simulink model "IIR4_int_quant"  (R2016b)
settings: Solver=VariableStepAuto  StartTime=0.0  StopTime=10.0  RelTol=1e-3
libraries: dspstat3 x2
settings Model: Creator=biren  LastModifiedBy=biren

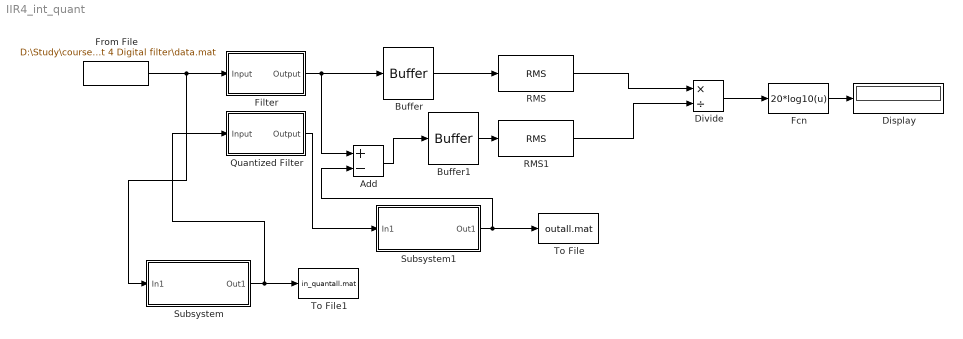
== system IIR4_int_quant ==
  Add : Sum  Inputs=+-
  Buffer : Buffer  TreatMby1Signals=One channel  OutputFrames=off
  Buffer1 : Buffer  TreatMby1Signals=One channel  OutputFrames=off
  Display : Display
  Divide : Product  Inputs=*/
  Fcn : Fcn  Expr=20*log10(u)
  "Filter " : Subsystem  Tag=FilterWizardSubSystem
      settings: ErrorFcn=dspFilterRealizedInBasicElemsAlgLoopErrFcnCallback
  From File : FromFile  FileName=D:\Study\courses\ECEN654\Assignment 4 Digital filter\data.mat  SampleTime=1/44100
  Quantized Filter : Subsystem  Tag=FilterWizardSubSystem  mask{ck=11}
      settings: ErrorFcn=dspFilterRealizedInBasicElemsAlgLoopErrFcnCallback
  RMS : dspstat3/RMS  run=off  directionMode=Each column  dimension=1  InputProcessing=Columns as channels (frame based)  reset_popup=None
  RMS1 : dspstat3/RMS  run=off  directionMode=Each column  dimension=1  InputProcessing=Columns as channels (frame based)  reset_popup=None
  Subsystem : Subsystem  mask{k=12, s=5}
  Subsystem1 : Subsystem  mask{k=12, s=5}
  To File : ToFile  Filename=outall.mat
  To File1 : ToFile  Filename=in_quantall.mat
  wires:
  "Filter "/1(Output) -> Buffer/1, Add/1
  Add/1 -> Buffer1/1
  Buffer/1 -> RMS/1
  Buffer1/1 -> RMS1/1
  Subsystem1/1(Out1) -> To File/1, Add/2
  Subsystem/1(Out1) -> To File1/1, Quantized Filter/1(Input)
  From File/1 -> Subsystem/1(In1), "Filter "/1(Input)
  RMS/1 -> Divide/1
  RMS1/1 -> Divide/2
  Divide/1 -> Fcn/1
  Fcn/1 -> Display/1
  Quantized Filter/1(Output) -> Subsystem1/1(In1)

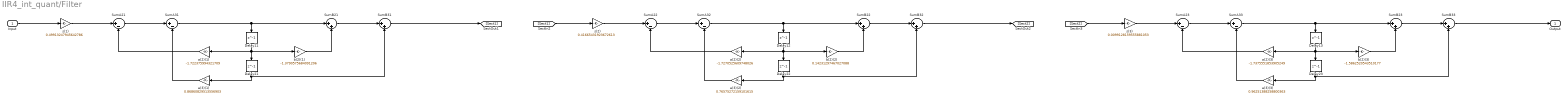
== system IIR4_int_quant/Filter  ==
  Input : Inport
  Delay{11..13,21..23} (6 alike) : Delay  DelayLength=1  InitialCondition=0
  SumA{21..23,31..33} (6 alike) : Sum  Inputs=|+-  RndMeth=Nearest  SaturateOnIntegerOverflow=on  OutDataTypeStr=Inherit: Same as first input
  SumB{21..23,31..33} (6 alike) : Sum  Inputs=|++  RndMeth=Nearest  SaturateOnIntegerOverflow=on  OutDataTypeStr=Inherit: Same as first input
  a(2)(1) : Gain  Gain=-1.722375994321709  ParamDataTypeStr=double  RndMeth=Nearest  SaturateOnIntegerOverflow=on  OutDataTypeStr=Inherit: Same as input
  a(2)(2) : Gain  Gain=-1.7270525609748026  ParamDataTypeStr=double  RndMeth=Nearest  SaturateOnIntegerOverflow=on  OutDataTypeStr=Inherit: Same as input
  a(2)(3) : Gain  Gain=-1.7375551853905249  ParamDataTypeStr=double  RndMeth=Nearest  SaturateOnIntegerOverflow=on  OutDataTypeStr=Inherit: Same as input
  a(3)(1) : Gain  Gain=0.86860829513556903  ParamDataTypeStr=double  RndMeth=Nearest  SaturateOnIntegerOverflow=on  OutDataTypeStr=Inherit: Same as input
  a(3)(2) : Gain  Gain=0.76575272159101615  ParamDataTypeStr=double  RndMeth=Nearest  SaturateOnIntegerOverflow=on  OutDataTypeStr=Inherit: Same as input
  a(3)(3) : Gain  Gain=0.96251388258800363  ParamDataTypeStr=double  RndMeth=Nearest  SaturateOnIntegerOverflow=on  OutDataTypeStr=Inherit: Same as input
  b(2)(1) : Gain  Gain=-1.3790575684091206  ParamDataTypeStr=double  RndMeth=Nearest  SaturateOnIntegerOverflow=on  OutDataTypeStr=Inherit: Same as input
  b(2)(2) : Gain  Gain=0.14231297467027088  ParamDataTypeStr=double  RndMeth=Nearest  SaturateOnIntegerOverflow=on  OutDataTypeStr=Inherit: Same as input
  b(2)(3) : Gain  Gain=-1.5862520543510177  ParamDataTypeStr=double  RndMeth=Nearest  SaturateOnIntegerOverflow=on  OutDataTypeStr=Inherit: Same as input
  s(1) : Gain  Gain=0.49913247945642786  ParamDataTypeStr=double  RndMeth=Nearest  SaturateOnIntegerOverflow=on  OutDataTypeStr=Inherit: Same as input
  s(2) : Gain  Gain=0.41665431923672613  ParamDataTypeStr=double  RndMeth=Nearest  SaturateOnIntegerOverflow=on  OutDataTypeStr=Inherit: Same as input
  s(3) : Gain  Gain=0.0099128159555881053  ParamDataTypeStr=double  RndMeth=Nearest  SaturateOnIntegerOverflow=on  OutDataTypeStr=Inherit: Same as input
  Output : Outport
  wires:
  Input/1 -> s(1)/1
  s(1)/1 -> SumA21/1
  SumA21/1 -> SumA31/1
  SumA31/1 -> SumB21/1, Delay11/1
  SumB21/1 -> SumB31/1
  SumB31/1 -> [Sect1]
  a(2)(1)/1 -> SumA21/2
  Delay11/1 -> a(2)(1)/1, b(2)(1)/1, Delay21/1
  b(2)(1)/1 -> SumB21/2
  a(3)(1)/1 -> SumA31/2
  Delay21/1 -> a(3)(1)/1, SumB31/2
  [Sect1] -> s(2)/1
  s(2)/1 -> SumA22/1
  SumA22/1 -> SumA32/1
  SumA32/1 -> SumB22/1, Delay12/1
  SumB22/1 -> SumB32/1
  SumB32/1 -> [Sect2]
  a(2)(2)/1 -> SumA22/2
  Delay12/1 -> a(2)(2)/1, b(2)(2)/1, Delay22/1
  b(2)(2)/1 -> SumB22/2
  a(3)(2)/1 -> SumA32/2
  Delay22/1 -> a(3)(2)/1, SumB32/2
  [Sect2] -> s(3)/1
  s(3)/1 -> SumA23/1
  SumA23/1 -> SumA33/1
  SumA33/1 -> SumB23/1, Delay13/1
  SumB23/1 -> SumB33/1
  SumB33/1 -> Output/1
  a(2)(3)/1 -> SumA23/2
  Delay13/1 -> a(2)(3)/1, b(2)(3)/1, Delay23/1
  b(2)(3)/1 -> SumB23/2
  a(3)(3)/1 -> SumA33/2
  Delay23/1 -> a(3)(3)/1, SumB33/2

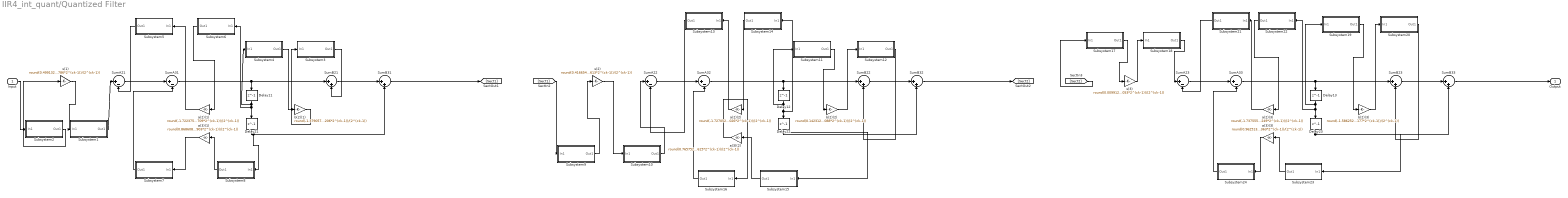
== system IIR4_int_quant/Quantized Filter ==
  Input : Inport
  Delay{11..13,21..23} (6 alike) : Delay  DelayLength=1  InitialCondition=0
  Subsystem1 : Subsystem  mask{k=12, s=5}
  Subsystem10 : Subsystem  mask{k=12, s=5}
  Subsystem11 : Subsystem  mask{k=12, s=5}
  Subsystem12 : Subsystem  mask{k=12, s=5}
  Subsystem13 : Subsystem  mask{k=12, s=5}
  Subsystem14 : Subsystem  mask{k=12, s=5}
  Subsystem15 : Subsystem  mask{k=12, s=5}
  Subsystem16 : Subsystem  mask{k=12, s=5}
  Subsystem17 : Subsystem  mask{k=12, s=5}
  Subsystem18 : Subsystem  mask{k=12, s=5}
  Subsystem19 : Subsystem  mask{k=12, s=5}
  Subsystem2 : Subsystem  mask{k=12, s=5}
  Subsystem20 : Subsystem  mask{k=12, s=5}
  Subsystem21 : Subsystem  mask{k=12, s=5}
  Subsystem22 : Subsystem  mask{k=12, s=5}
  Subsystem23 : Subsystem  mask{k=12, s=5}
  Subsystem24 : Subsystem  mask{k=12, s=5}
  Subsystem3 : Subsystem  mask{k=12, s=5}
  Subsystem4 : Subsystem  mask{k=12, s=5}
  Subsystem5 : Subsystem  mask{k=12, s=5}
  Subsystem6 : Subsystem  mask{k=12, s=5}
  Subsystem7 : Subsystem  mask{k=12, s=5}
  Subsystem8 : Subsystem  mask{k=12, s=5}
  Subsystem9 : Subsystem  mask{k=12, s=5}
  SumA{21..23,31..33} (6 alike) : Sum  Inputs=|+-  RndMeth=Nearest  SaturateOnIntegerOverflow=on  OutDataTypeStr=Inherit: Same as first input
  SumB{21..23,31..33} (6 alike) : Sum  Inputs=|++  RndMeth=Nearest  SaturateOnIntegerOverflow=on  OutDataTypeStr=Inherit: Same as first input
  a(2)(1) : Gain  Gain=round(-1.722375994321709*2^(ck-1))/(2^(ck-1))  ParamDataTypeStr=double  RndMeth=Nearest  SaturateOnIntegerOverflow=on  OutDataTypeStr=Inherit: Same as input
  a(2)(2) : Gain  Gain=round(-1.7270525609748026*2^(ck-1))/(2^(ck-1))  ParamDataTypeStr=double  RndMeth=Nearest  SaturateOnIntegerOverflow=on  OutDataTypeStr=Inherit: Same as input
  a(2)(3) : Gain  Gain=round(-1.7375551853905249*2^(ck-1))/(2^(ck-1))  ParamDataTypeStr=double  RndMeth=Nearest  SaturateOnIntegerOverflow=on  OutDataTypeStr=Inherit: Same as input
  a(3)(1) : Gain  Gain=round(0.86860829513556903*2^(ck-1))/(2^(ck-1))  ParamDataTypeStr=double  RndMeth=Nearest  SaturateOnIntegerOverflow=on  OutDataTypeStr=Inherit: Same as input
  a(3)(2) : Gain  Gain=round(0.76575272159101615*2^(ck-1))/(2^(ck-1))  ParamDataTypeStr=double  RndMeth=Nearest  SaturateOnIntegerOverflow=on  OutDataTypeStr=Inherit: Same as input
  a(3)(3) : Gain  Gain=round(0.96251388258800363*2^(ck-1))/(2^(ck-1))  ParamDataTypeStr=double  RndMeth=Nearest  SaturateOnIntegerOverflow=on  OutDataTypeStr=Inherit: Same as input
  b(2)(1) : Gain  Gain=round(-1.3790575684091206*2^(ck-1))/(2^(ck-1))  ParamDataTypeStr=double  RndMeth=Nearest  SaturateOnIntegerOverflow=on  OutDataTypeStr=Inherit: Same as input
  b(2)(2) : Gain  Gain=round(0.14231297467027088*2^(ck-1))/(2^(ck-1))  ParamDataTypeStr=double  RndMeth=Nearest  SaturateOnIntegerOverflow=on  OutDataTypeStr=Inherit: Same as input
  b(2)(3) : Gain  Gain=round(-1.5862520543510177*2^(ck-1))/(2^(ck-1))  ParamDataTypeStr=double  RndMeth=Nearest  SaturateOnIntegerOverflow=on  OutDataTypeStr=Inherit: Same as input
  s(1) : Gain  Gain=round(0.49913247945642786*2^(ck-1))/(2^(ck-1))  ParamDataTypeStr=double  RndMeth=Nearest  SaturateOnIntegerOverflow=on  OutDataTypeStr=Inherit: Same as input
  s(2) : Gain  Gain=round(0.41665431923672613*2^(ck-1))/(2^(ck-1))  ParamDataTypeStr=double  RndMeth=Nearest  SaturateOnIntegerOverflow=on  OutDataTypeStr=Inherit: Same as input
  s(3) : Gain  Gain=round(0.0099128159555881053*2^(ck-1))/(2^(ck-1))  ParamDataTypeStr=double  RndMeth=Nearest  SaturateOnIntegerOverflow=on  OutDataTypeStr=Inherit: Same as input
  Output : Outport
  wires:
  SumA21/1 -> SumA31/1
  SumA31/1 -> SumB21/1, Delay11/1
  SumB21/1 -> SumB31/1
  SumB31/1 -> [Sect1]
  Delay11/1 -> Subsystem4/1(In1), Subsystem6/1(In1), Delay21/1
  Delay21/1 -> Subsystem8/1(In1), SumB31/2
  SumA22/1 -> SumA32/1
  SumA32/1 -> SumB22/1, Delay12/1
  SumB22/1 -> SumB32/1
  SumB32/1 -> [Sect2]
  Delay12/1 -> Subsystem11/1(In1), Subsystem14/1(In1), Delay22/1
  Delay22/1 -> Subsystem15/1(In1), SumB32/2
  SumA23/1 -> SumA33/1
  SumA33/1 -> SumB23/1, Delay13/1
  SumB23/1 -> SumB33/1
  SumB33/1 -> Output/1
  Delay13/1 -> Subsystem19/1(In1), Subsystem22/1(In1), Delay23/1
  Delay23/1 -> Subsystem23/1(In1), SumB33/2
  s(1)/1 -> Subsystem1/1(In1)
  Subsystem1/1(Out1) -> SumA21/1
  Input/1 -> Subsystem2/1(In1)
  Subsystem2/1(Out1) -> s(1)/1
  Subsystem4/1(Out1) -> b(2)(1)/1
  b(2)(1)/1 -> Subsystem3/1(In1)
  Subsystem3/1(Out1) -> SumB21/2
  Subsystem6/1(Out1) -> a(2)(1)/1
  a(2)(1)/1 -> Subsystem5/1(In1)
  Subsystem5/1(Out1) -> SumA21/2
  Subsystem8/1(Out1) -> a(3)(1)/1
  a(3)(1)/1 -> Subsystem7/1(In1)
  Subsystem7/1(Out1) -> SumA31/2
  [Sect1] -> Subsystem9/1(In1)
  Subsystem9/1(Out1) -> s(2)/1
  s(2)/1 -> Subsystem10/1(In1)
  Subsystem10/1(Out1) -> SumA22/1
  Subsystem11/1(Out1) -> b(2)(2)/1
  b(2)(2)/1 -> Subsystem12/1(In1)
  Subsystem12/1(Out1) -> SumB22/2
  Subsystem14/1(Out1) -> a(2)(2)/1
  a(2)(2)/1 -> Subsystem13/1(In1)
  Subsystem13/1(Out1) -> SumA22/2
  Subsystem15/1(Out1) -> a(3)(2)/1
  a(3)(2)/1 -> Subsystem16/1(In1)
  Subsystem16/1(Out1) -> SumA32/2
  [Sect2] -> Subsystem17/1(In1)
  Subsystem17/1(Out1) -> s(3)/1
  s(3)/1 -> Subsystem18/1(In1)
  Subsystem18/1(Out1) -> SumA23/1
  Subsystem19/1(Out1) -> b(2)(3)/1
  b(2)(3)/1 -> Subsystem20/1(In1)
  Subsystem20/1(Out1) -> SumB23/2
  Subsystem22/1(Out1) -> a(2)(3)/1
  a(2)(3)/1 -> Subsystem21/1(In1)
  Subsystem21/1(Out1) -> SumA23/2
  Subsystem23/1(Out1) -> a(3)(3)/1
  Subsystem24/1(Out1) -> SumA33/2
  a(3)(3)/1 -> Subsystem24/1(In1)

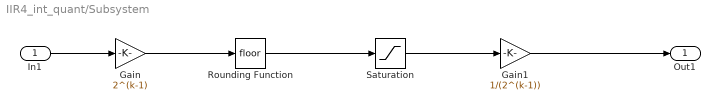
== system IIR4_int_quant/Subsystem ==
  In1 : Inport
  Gain : Gain  Gain=2^(k-1)
  Gain1 : Gain  Gain=1/(2^(k-1))
  Rounding Function : Rounding
  Saturation : Saturate  UpperLimit=2^(k+s-1) - 1  LowerLimit=-2^(k+s-1)
  Out1 : Outport
  wires:
  In1/1 -> Gain/1
  Gain/1 -> Rounding Function/1
  Rounding Function/1 -> Saturation/1
  Saturation/1 -> Gain1/1
  Gain1/1 -> Out1/1

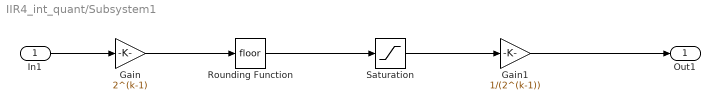
== system IIR4_int_quant/Subsystem1 ==
  In1 : Inport
  Gain : Gain  Gain=2^(k-1)
  Gain1 : Gain  Gain=1/(2^(k-1))
  Rounding Function : Rounding
  Saturation : Saturate  UpperLimit=2^(k+s-1) - 1  LowerLimit=-2^(k+s-1)
  Out1 : Outport
  wires:
  In1/1 -> Gain/1
  Gain/1 -> Rounding Function/1
  Rounding Function/1 -> Saturation/1
  Saturation/1 -> Gain1/1
  Gain1/1 -> Out1/1

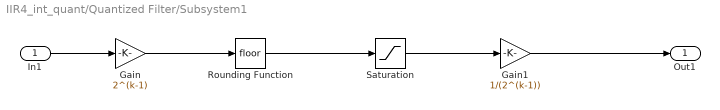
== system IIR4_int_quant/Quantized Filter/Subsystem1 ==
  In1 : Inport
  Gain : Gain  Gain=2^(k-1)
  Gain1 : Gain  Gain=1/(2^(k-1))
  Rounding Function : Rounding
  Saturation : Saturate  UpperLimit=2^(k+s-1) - 1  LowerLimit=-2^(k+s-1)
  Out1 : Outport
  wires:
  In1/1 -> Gain/1
  Gain/1 -> Rounding Function/1
  Rounding Function/1 -> Saturation/1
  Saturation/1 -> Gain1/1
  Gain1/1 -> Out1/1

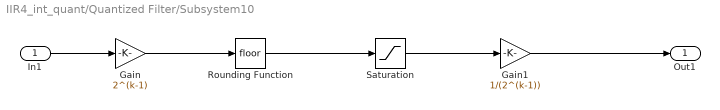
== system IIR4_int_quant/Quantized Filter/Subsystem10 ==
  In1 : Inport
  Gain : Gain  Gain=2^(k-1)
  Gain1 : Gain  Gain=1/(2^(k-1))
  Rounding Function : Rounding
  Saturation : Saturate  UpperLimit=2^(k+s-1) - 1  LowerLimit=-2^(k+s-1)
  Out1 : Outport
  wires:
  In1/1 -> Gain/1
  Gain/1 -> Rounding Function/1
  Rounding Function/1 -> Saturation/1
  Saturation/1 -> Gain1/1
  Gain1/1 -> Out1/1

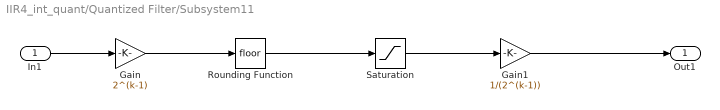
== system IIR4_int_quant/Quantized Filter/Subsystem11 ==
  In1 : Inport
  Gain : Gain  Gain=2^(k-1)
  Gain1 : Gain  Gain=1/(2^(k-1))
  Rounding Function : Rounding
  Saturation : Saturate  UpperLimit=2^(k+s-1) - 1  LowerLimit=-2^(k+s-1)
  Out1 : Outport
  wires:
  In1/1 -> Gain/1
  Gain/1 -> Rounding Function/1
  Rounding Function/1 -> Saturation/1
  Saturation/1 -> Gain1/1
  Gain1/1 -> Out1/1

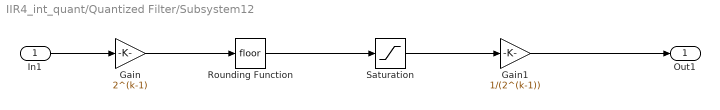
== system IIR4_int_quant/Quantized Filter/Subsystem12 ==
  In1 : Inport
  Gain : Gain  Gain=2^(k-1)
  Gain1 : Gain  Gain=1/(2^(k-1))
  Rounding Function : Rounding
  Saturation : Saturate  UpperLimit=2^(k+s-1) - 1  LowerLimit=-2^(k+s-1)
  Out1 : Outport
  wires:
  In1/1 -> Gain/1
  Gain/1 -> Rounding Function/1
  Rounding Function/1 -> Saturation/1
  Saturation/1 -> Gain1/1
  Gain1/1 -> Out1/1

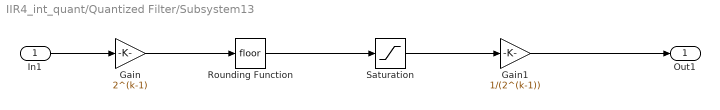
== system IIR4_int_quant/Quantized Filter/Subsystem13 ==
  In1 : Inport
  Gain : Gain  Gain=2^(k-1)
  Gain1 : Gain  Gain=1/(2^(k-1))
  Rounding Function : Rounding
  Saturation : Saturate  UpperLimit=2^(k+s-1) - 1  LowerLimit=-2^(k+s-1)
  Out1 : Outport
  wires:
  In1/1 -> Gain/1
  Gain/1 -> Rounding Function/1
  Rounding Function/1 -> Saturation/1
  Saturation/1 -> Gain1/1
  Gain1/1 -> Out1/1

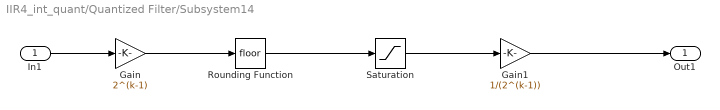
== system IIR4_int_quant/Quantized Filter/Subsystem14 ==
  In1 : Inport
  Gain : Gain  Gain=2^(k-1)
  Gain1 : Gain  Gain=1/(2^(k-1))
  Rounding Function : Rounding
  Saturation : Saturate  UpperLimit=2^(k+s-1) - 1  LowerLimit=-2^(k+s-1)
  Out1 : Outport
  wires:
  In1/1 -> Gain/1
  Gain/1 -> Rounding Function/1
  Rounding Function/1 -> Saturation/1
  Saturation/1 -> Gain1/1
  Gain1/1 -> Out1/1

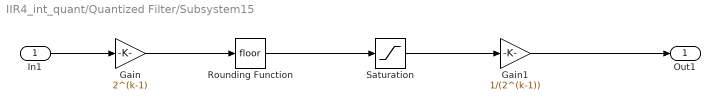
== system IIR4_int_quant/Quantized Filter/Subsystem15 ==
  In1 : Inport
  Gain : Gain  Gain=2^(k-1)
  Gain1 : Gain  Gain=1/(2^(k-1))
  Rounding Function : Rounding
  Saturation : Saturate  UpperLimit=2^(k+s-1) - 1  LowerLimit=-2^(k+s-1)
  Out1 : Outport
  wires:
  In1/1 -> Gain/1
  Gain/1 -> Rounding Function/1
  Rounding Function/1 -> Saturation/1
  Saturation/1 -> Gain1/1
  Gain1/1 -> Out1/1

== system IIR4_int_quant/Quantized Filter/Subsystem16 ==
  In1 : Inport
  Gain : Gain  Gain=2^(k-1)
  Gain1 : Gain  Gain=1/(2^(k-1))
  Rounding Function : Rounding
  Saturation : Saturate  UpperLimit=2^(k+s-1) - 1  LowerLimit=-2^(k+s-1)
  Out1 : Outport
  wires:
  In1/1 -> Gain/1
  Gain/1 -> Rounding Function/1
  Rounding Function/1 -> Saturation/1
  Saturation/1 -> Gain1/1
  Gain1/1 -> Out1/1

== system IIR4_int_quant/Quantized Filter/Subsystem17 ==
  In1 : Inport
  Gain : Gain  Gain=2^(k-1)
  Gain1 : Gain  Gain=1/(2^(k-1))
  Rounding Function : Rounding
  Saturation : Saturate  UpperLimit=2^(k+s-1) - 1  LowerLimit=-2^(k+s-1)
  Out1 : Outport
  wires:
  In1/1 -> Gain/1
  Gain/1 -> Rounding Function/1
  Rounding Function/1 -> Saturation/1
  Saturation/1 -> Gain1/1
  Gain1/1 -> Out1/1

== system IIR4_int_quant/Quantized Filter/Subsystem18 ==
  In1 : Inport
  Gain : Gain  Gain=2^(k-1)
  Gain1 : Gain  Gain=1/(2^(k-1))
  Rounding Function : Rounding
  Saturation : Saturate  UpperLimit=2^(k+s-1) - 1  LowerLimit=-2^(k+s-1)
  Out1 : Outport
  wires:
  In1/1 -> Gain/1
  Gain/1 -> Rounding Function/1
  Rounding Function/1 -> Saturation/1
  Saturation/1 -> Gain1/1
  Gain1/1 -> Out1/1

== system IIR4_int_quant/Quantized Filter/Subsystem19 ==
  In1 : Inport
  Gain : Gain  Gain=2^(k-1)
  Gain1 : Gain  Gain=1/(2^(k-1))
  Rounding Function : Rounding
  Saturation : Saturate  UpperLimit=2^(k+s-1) - 1  LowerLimit=-2^(k+s-1)
  Out1 : Outport
  wires:
  In1/1 -> Gain/1
  Gain/1 -> Rounding Function/1
  Rounding Function/1 -> Saturation/1
  Saturation/1 -> Gain1/1
  Gain1/1 -> Out1/1

== system IIR4_int_quant/Quantized Filter/Subsystem2 ==
  In1 : Inport
  Gain : Gain  Gain=2^(k-1)
  Gain1 : Gain  Gain=1/(2^(k-1))
  Rounding Function : Rounding
  Saturation : Saturate  UpperLimit=2^(k+s-1) - 1  LowerLimit=-2^(k+s-1)
  Out1 : Outport
  wires:
  In1/1 -> Gain/1
  Gain/1 -> Rounding Function/1
  Rounding Function/1 -> Saturation/1
  Saturation/1 -> Gain1/1
  Gain1/1 -> Out1/1

== system IIR4_int_quant/Quantized Filter/Subsystem20 ==
  In1 : Inport
  Gain : Gain  Gain=2^(k-1)
  Gain1 : Gain  Gain=1/(2^(k-1))
  Rounding Function : Rounding
  Saturation : Saturate  UpperLimit=2^(k+s-1) - 1  LowerLimit=-2^(k+s-1)
  Out1 : Outport
  wires:
  In1/1 -> Gain/1
  Gain/1 -> Rounding Function/1
  Rounding Function/1 -> Saturation/1
  Saturation/1 -> Gain1/1
  Gain1/1 -> Out1/1

== system IIR4_int_quant/Quantized Filter/Subsystem21 ==
  In1 : Inport
  Gain : Gain  Gain=2^(k-1)
  Gain1 : Gain  Gain=1/(2^(k-1))
  Rounding Function : Rounding
  Saturation : Saturate  UpperLimit=2^(k+s-1) - 1  LowerLimit=-2^(k+s-1)
  Out1 : Outport
  wires:
  In1/1 -> Gain/1
  Gain/1 -> Rounding Function/1
  Rounding Function/1 -> Saturation/1
  Saturation/1 -> Gain1/1
  Gain1/1 -> Out1/1

== system IIR4_int_quant/Quantized Filter/Subsystem22 ==
  In1 : Inport
  Gain : Gain  Gain=2^(k-1)
  Gain1 : Gain  Gain=1/(2^(k-1))
  Rounding Function : Rounding
  Saturation : Saturate  UpperLimit=2^(k+s-1) - 1  LowerLimit=-2^(k+s-1)
  Out1 : Outport
  wires:
  In1/1 -> Gain/1
  Gain/1 -> Rounding Function/1
  Rounding Function/1 -> Saturation/1
  Saturation/1 -> Gain1/1
  Gain1/1 -> Out1/1

== system IIR4_int_quant/Quantized Filter/Subsystem23 ==
  In1 : Inport
  Gain : Gain  Gain=2^(k-1)
  Gain1 : Gain  Gain=1/(2^(k-1))
  Rounding Function : Rounding
  Saturation : Saturate  UpperLimit=2^(k+s-1) - 1  LowerLimit=-2^(k+s-1)
  Out1 : Outport
  wires:
  In1/1 -> Gain/1
  Gain/1 -> Rounding Function/1
  Rounding Function/1 -> Saturation/1
  Saturation/1 -> Gain1/1
  Gain1/1 -> Out1/1

== system IIR4_int_quant/Quantized Filter/Subsystem24 ==
  In1 : Inport
  Gain : Gain  Gain=2^(k-1)
  Gain1 : Gain  Gain=1/(2^(k-1))
  Rounding Function : Rounding
  Saturation : Saturate  UpperLimit=2^(k+s-1) - 1  LowerLimit=-2^(k+s-1)
  Out1 : Outport
  wires:
  In1/1 -> Gain/1
  Gain/1 -> Rounding Function/1
  Rounding Function/1 -> Saturation/1
  Saturation/1 -> Gain1/1
  Gain1/1 -> Out1/1

== system IIR4_int_quant/Quantized Filter/Subsystem3 ==
  In1 : Inport
  Gain : Gain  Gain=2^(k-1)
  Gain1 : Gain  Gain=1/(2^(k-1))
  Rounding Function : Rounding
  Saturation : Saturate  UpperLimit=2^(k+s-1) - 1  LowerLimit=-2^(k+s-1)
  Out1 : Outport
  wires:
  In1/1 -> Gain/1
  Gain/1 -> Rounding Function/1
  Rounding Function/1 -> Saturation/1
  Saturation/1 -> Gain1/1
  Gain1/1 -> Out1/1

== system IIR4_int_quant/Quantized Filter/Subsystem4 ==
  In1 : Inport
  Gain : Gain  Gain=2^(k-1)
  Gain1 : Gain  Gain=1/(2^(k-1))
  Rounding Function : Rounding
  Saturation : Saturate  UpperLimit=2^(k+s-1) - 1  LowerLimit=-2^(k+s-1)
  Out1 : Outport
  wires:
  In1/1 -> Gain/1
  Gain/1 -> Rounding Function/1
  Rounding Function/1 -> Saturation/1
  Saturation/1 -> Gain1/1
  Gain1/1 -> Out1/1

== system IIR4_int_quant/Quantized Filter/Subsystem5 ==
  In1 : Inport
  Gain : Gain  Gain=2^(k-1)
  Gain1 : Gain  Gain=1/(2^(k-1))
  Rounding Function : Rounding
  Saturation : Saturate  UpperLimit=2^(k+s-1) - 1  LowerLimit=-2^(k+s-1)
  Out1 : Outport
  wires:
  In1/1 -> Gain/1
  Gain/1 -> Rounding Function/1
  Rounding Function/1 -> Saturation/1
  Saturation/1 -> Gain1/1
  Gain1/1 -> Out1/1

== system IIR4_int_quant/Quantized Filter/Subsystem6 ==
  In1 : Inport
  Gain : Gain  Gain=2^(k-1)
  Gain1 : Gain  Gain=1/(2^(k-1))
  Rounding Function : Rounding
  Saturation : Saturate  UpperLimit=2^(k+s-1) - 1  LowerLimit=-2^(k+s-1)
  Out1 : Outport
  wires:
  In1/1 -> Gain/1
  Gain/1 -> Rounding Function/1
  Rounding Function/1 -> Saturation/1
  Saturation/1 -> Gain1/1
  Gain1/1 -> Out1/1

== system IIR4_int_quant/Quantized Filter/Subsystem7 ==
  In1 : Inport
  Gain : Gain  Gain=2^(k-1)
  Gain1 : Gain  Gain=1/(2^(k-1))
  Rounding Function : Rounding
  Saturation : Saturate  UpperLimit=2^(k+s-1) - 1  LowerLimit=-2^(k+s-1)
  Out1 : Outport
  wires:
  In1/1 -> Gain/1
  Gain/1 -> Rounding Function/1
  Rounding Function/1 -> Saturation/1
  Saturation/1 -> Gain1/1
  Gain1/1 -> Out1/1

== system IIR4_int_quant/Quantized Filter/Subsystem8 ==
  In1 : Inport
  Gain : Gain  Gain=2^(k-1)
  Gain1 : Gain  Gain=1/(2^(k-1))
  Rounding Function : Rounding
  Saturation : Saturate  UpperLimit=2^(k+s-1) - 1  LowerLimit=-2^(k+s-1)
  Out1 : Outport
  wires:
  In1/1 -> Gain/1
  Gain/1 -> Rounding Function/1
  Rounding Function/1 -> Saturation/1
  Saturation/1 -> Gain1/1
  Gain1/1 -> Out1/1

== system IIR4_int_quant/Quantized Filter/Subsystem9 ==
  In1 : Inport
  Gain : Gain  Gain=2^(k-1)
  Gain1 : Gain  Gain=1/(2^(k-1))
  Rounding Function : Rounding
  Saturation : Saturate  UpperLimit=2^(k+s-1) - 1  LowerLimit=-2^(k+s-1)
  Out1 : Outport
  wires:
  In1/1 -> Gain/1
  Gain/1 -> Rounding Function/1
  Rounding Function/1 -> Saturation/1
  Saturation/1 -> Gain1/1
  Gain1/1 -> Out1/1
